simulink model "RefModel_SystemArchitecture"  (R2020a)
settings: Solver=ode1  StartTime=0.0  StopTime=inf  FixedStep=Ts_BigModel.Ts_base  MaxStep=Ts  RelTol=1e-3
undefined symbols (not defined in the file or in its folder): airspeed1, ENUM_SystemHealthStatus, ENUM_UavModel_Architecture, radar1, TASK_SET
libraries: simulink x1
settings Model: Creator=sl  LastModifiedBy=Administrator
settings DataIOCC: SaveOutput=off  SaveTime=off
settings OptimizationCC: DefaultParameterBehavior=Inlined  EnhancedBackFolding=on  PassReuseOutputArgsAs=Individual arguments  ZeroExternalMemoryAtStartup=off  ZeroInternalMemoryAtStartup=off  OptimizeBlockOrder=speed  DifferentSizesBufferReuse=on  OptimizationCustomize=off  EfficientTunableParamExpr=on
settings DebuggingCC: InheritedTsInSrcMsg=none  ParameterPrecisionLossMsg=none  ParameterTunabilityLossMsg=error  UnconnectedInputMsg=none  UnconnectedOutputMsg=none  UnconnectedLineMsg=none
settings HardwareCC: ProdBitPerPointer=32  ProdBitPerSizeT=32  ProdBitPerPtrDiffT=32  ProdLargestAtomicInteger=Long  ProdLargestAtomicFloat=Double  ProdWordSize=32  ProdHWDeviceType=ARM Compatible->ARM Cortex
settings ModelReferenceCC: ParallelModelReferenceMATLABWorkerInit=Copy Base Workspace  ModelReferenceNumInstancesAllowed=Single
settings SFSimCC: MATLABDynamicMemAlloc=off
settings RTWCC: SystemTargetFile=ert.tlc  GenCodeOnly=on  PackageGeneratedCodeAndArtifacts=on  TemplateMakefile=ert_default_tmf  GenerateReport=on  IncludeHyperlinkInReport=on  LaunchReport=on  GenerateTraceInfo=on  GenerateTraceReport=on  GenerateTraceReportSl=on  GenerateTraceReportSf=on  GenerateTraceReportEml=on
settings CodeAppCC: ForceParamTrailComments=on  IgnoreCustomStorageClasses=off  MaxIdLength=48  OperatorAnnotations=on  SimulinkDataObjDesc=on  SFDataObjDesc=on  MATLABFcnDesc=on  InsertBlockDesc=on  MATLABSourceComments=on
settings ERTTargetCC: TargetLangStandard=C99 (ISO)  GenerateSampleERTMain=on  LogVarNameModifier=none  SupportVariableSizeSignals=on  InlinedParameterPlacement=NonHierarchical  ERTCustomFileTemplate=example_file_process.tlc  ERTFilePackagingFormat=Compact

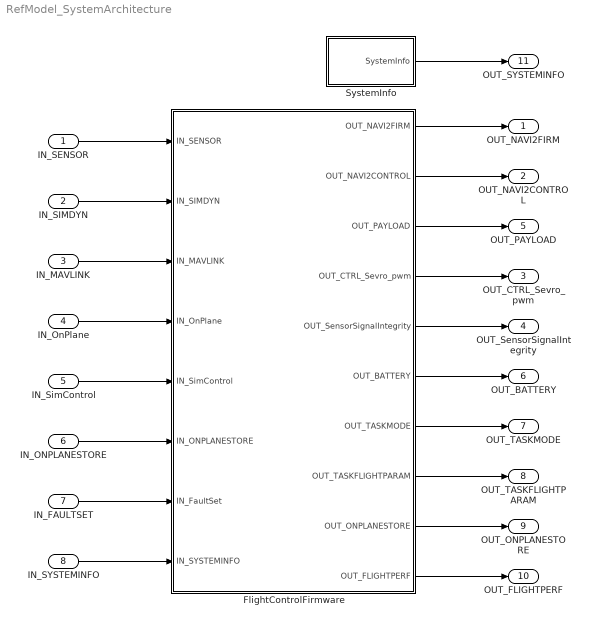
== system RefModel_SystemArchitecture ==
  IN_SENSOR : Inport  OutDataTypeStr=Bus: BUS_SENSOR
  IN_SIMDYN : Inport  Port=2  OutDataTypeStr=Bus: BUS_UAVDYN_FlightParam
  IN_MAVLINK : Inport  Port=3  OutDataTypeStr=Bus: BUS_MAVLINK_TO_FIRM  BusOutputAsStruct=on
  IN_OnPlane : Inport  Port=4  OutDataTypeStr=Bus: BUS_ONPLANE_FEEDBACK  BusOutputAsStruct=on
  IN_SimControl : Inport  Port=5  OutDataTypeStr=Bus: BUS_SIMCONTROL  BusOutputAsStruct=on
  IN_ONPLANESTORE : Inport  Port=6  OutDataTypeStr=Bus: BUS_ONPLANE_STORE  BusOutputAsStruct=on
  IN_FAULTSET : Inport  Port=7  OutDataTypeStr=Bus: BUS_SENSORFAULT_IN  BusOutputAsStruct=on
  IN_SYSTEMINFO : Inport  Port=8  OutDataTypeStr=Bus: BUS_SYSTEMINFO_INPUT  BusOutputAsStruct=on
  FlightControlFirmware : Subsystem
  SystemInfo : Subsystem
  " OUT_NAVI2FIRM" : Outport  OutDataTypeStr=Bus: BUS_NAVI_TO_FIRM
  OUT_NAVI2CONTROL : Outport  Port=2  OutDataTypeStr=Bus: BUS_TO_CONTROL
  OUT_CTRL_Sevro_pwm : Outport  Port=3  OutDataTypeStr=Bus: BUS_CTRL_Sevro_pwm  BusOutputAsStruct=on
  OUT_SensorSignalIntegrity : Outport  Port=4  OutDataTypeStr=Bus: BUS_NAVI_SensorSignalIntegrity
  OUT_PAYLOAD : Outport  Port=5  OutDataTypeStr=Bus: BUS_TASK_PAYLOAD  BusOutputAsStruct=on
  OUT_BATTERY : Outport  Port=6  OutDataTypeStr=Bus: BUS_TASK_BATTERY  BusOutputAsStruct=on
  OUT_TASKMODE : Outport  Port=7  OutDataTypeStr=Bus: BUS_TASK_PATH_OutParam
  OUT_TASKFLIGHTPARAM : Outport  Port=8  OutDataTypeStr=Bus: BUS_TASK_COMMON_OutParam
  OUT_ONPLANESTORE : Outport  Port=9  OutDataTypeStr=Bus: BUS_ONPLANE_STORE  BusOutputAsStruct=on
  OUT_FLIGHTPERF : Outport  Port=10  OutDataTypeStr=Bus: BUS_FLIGHTPERF_OUT
  " OUT_SYSTEMINFO" : Outport  Port=11  OutDataTypeStr=Bus: BUS_SYSTEMINFO  PortDimensions=1
  wires:
  IN_SIMDYN/1 -> FlightControlFirmware/2(IN_SIMDYN)
  FlightControlFirmware/4(OUT_CTRL_Sevro_pwm) -> OUT_CTRL_Sevro_pwm/1
  FlightControlFirmware/5(OUT_SensorSignalIntegrity) -> OUT_SensorSignalIntegrity/1
  FlightControlFirmware/1(OUT_NAVI2FIRM) -> " OUT_NAVI2FIRM"/1
  IN_OnPlane/1 -> FlightControlFirmware/4(IN_OnPlane)
  FlightControlFirmware/2(OUT_NAVI2CONTROL) -> OUT_NAVI2CONTROL/1
  IN_MAVLINK/1 -> FlightControlFirmware/3(IN_MAVLINK)
  FlightControlFirmware/3(OUT_PAYLOAD) -> OUT_PAYLOAD/1
  IN_SENSOR/1 -> FlightControlFirmware/1(IN_SENSOR)
  FlightControlFirmware/8(OUT_TASKFLIGHTPARAM) -> OUT_TASKFLIGHTPARAM/1
  FlightControlFirmware/7(OUT_TASKMODE) -> OUT_TASKMODE/1
  FlightControlFirmware/6(OUT_BATTERY) -> OUT_BATTERY/1
  IN_SimControl/1 -> FlightControlFirmware/5(IN_SimControl)
  IN_ONPLANESTORE/1 -> FlightControlFirmware/6(IN_ONPLANESTORE)
  FlightControlFirmware/9(OUT_ONPLANESTORE) -> OUT_ONPLANESTORE/1
  FlightControlFirmware/10(OUT_FLIGHTPERF) -> OUT_FLIGHTPERF/1
  IN_FAULTSET/1 -> FlightControlFirmware/7(IN_FaultSet)
  SystemInfo/1(SystemInfo) -> " OUT_SYSTEMINFO"/1
  IN_SYSTEMINFO/1 -> FlightControlFirmware/8(IN_SYSTEMINFO)

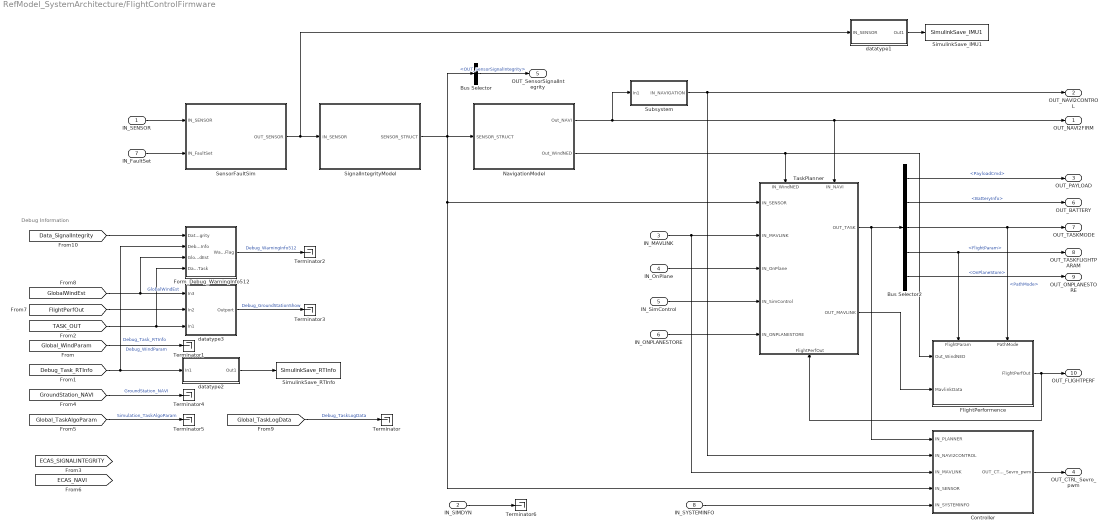
== system RefModel_SystemArchitecture/FlightControlFirmware ==
  note: Debug Information
  IN_SENSOR : Inport
  IN_SIMDYN : Inport  Port=2
  IN_MAVLINK : Inport  Port=3
  IN_OnPlane : Inport  Port=4
  IN_SimControl : Inport  Port=5
  IN_ONPLANESTORE : Inport  Port=6
  IN_FaultSet : Inport  Port=7
  IN_SYSTEMINFO : Inport  Port=8
  Bus Selector : BusSelector  OutputSignals=OUT_SensorSignalIntegrity
  Bus Selector2 : BusSelector  OutputSignals=PayloadCmd,BatteryInfo,PathMode,FlightParam,OnPlaneStore
  Controller : Subsystem
  FlightPerformence : Subsystem
      settings: PortSchema="{\"entries\":[{\"content\":{\"sides\":[{\"content\":{\"connectorIds\":[\"In1\",\"In2\"]},\"type\":\"ConnectorPlacement.EquallySpacedRectSide\",\"uuid\":\"433a6f53-ed4f-43c9-a2db-a1305bc564ee\"},{\"content\":{\"connectorIds\":[\"Out1\"],\"side\":\"RIGHT\"},\"type\":\"ConnectorPlacement.EquallySpacedRectSide\",\"uuid\":\"57435a5e-a27f-4849-b093-9cb5d83dc104\"},{\"content\":{\"connectorIds\":[\"In3\",\"In4\"],\"side\":\"TOP\"},\"type\":\"ConnectorPlacement.EquallySpacedRectSide\",\"uuid\":\"dceb23ba-b060-4a02-979b-0122130a3797\"}]},\"type\":\"ConnectorPlacement.EquallySpacedConnector\",\"uuid\":\"2c013d7c-89f2-45e4-826c-b5a23ebc63f7\"}],\"packageUris\":[\"http://schema.mathworks.com/mf0/Connector/19700101\"],\"version\":\"1.0\"}"
  Form_Debug_WarningInfo512 : Subsystem
  NavigationModel : Subsystem
  SensorFaultSim : Subsystem
  SignalIntegrityModel : Subsystem
  SimulinkSave_IMU1 : ToWorkspace  VariableName=SimulinkSave_IMU1  SaveFormat=Structure With Time  SampleTime=-1
  SimulinkSave_RTInfo : ToWorkspace  VariableName=SimulinkSave_RTInfo  SaveFormat=Structure With Time  SampleTime=-1
  Subsystem : Subsystem
  TaskPlanner : Subsystem
      settings: PortSchema="{\"entries\":[{\"content\":{\"sides\":[{\"content\":{\"connectorIds\":[\"In1\",\"In2\",\"In3\",\"In4\",\"In5\"]},\"type\":\"ConnectorPlacement.EquallySpacedRectSide\",\"uuid\":\"cf788447-cee3-4dc7-a19e-d1c3b675d866\"},{\"content\":{\"connectorIds\":[\"Out1\",\"Out2\"],\"side\":\"RIGHT\"},\"type\":\"ConnectorPlacement.EquallySpacedRectSide\",\"uuid\":\"de502817-2f17-4bc5-82c1-7b7d96fa5a18\"},{\"content\":{\"connectorIds\":[\"In6\",\"In7\"],\"side\":\"TOP\"},\"type\":\"ConnectorPlacement.EquallySpacedRectSide\",\"uuid\":\"c2c5d609-21c0-4e27-8129-13e054f6685c\"},{\"content\":{\"connectorIds\":[\"In8\"],\"side\":\"BOTTOM\"},\"type\":\"ConnectorPlacement.EquallySpacedRectSide\",\"uuid\":\"4fcd6bd9-9831-4959-9cb5-0a694e5ed564\"}]},\"type\":\"ConnectorPlacement.EquallySpacedConnector\",\"uuid\":\"8f2d23fd-8a63-42f8-87e9-439a9ee38a82\"}],\"packageUris\":[\"http://schema.mathworks.com/mf0/Connector/19700101\"],\"version\":\"1.0\"}"
  Terminator{,1..6} (7 alike) : Terminator
  datatype1 : Subsystem
  datatype2 : Subsystem
  datatype3 : Subsystem
  OUT_NAVI2FIRM : Outport
  OUT_NAVI2CONTROL : Outport  Port=2
  OUT_PAYLOAD : Outport  Port=3
  OUT_CTRL_Sevro_pwm : Outport  Port=4
  OUT_SensorSignalIntegrity : Outport  Port=5  OutDataTypeStr=Bus: BUS_NAVI_SensorSignalIntegrity
  OUT_BATTERY : Outport  Port=6
  OUT_TASKMODE : Outport  Port=7
  OUT_TASKFLIGHTPARAM : Outport  Port=8
  OUT_ONPLANESTORE : Outport  Port=9
  OUT_FLIGHTPERF : Outport  Port=10
  wires:
  Subsystem/1(IN_NAVIGATION) -> Controller/2(IN_NAVI2CONTROL), OUT_NAVI2CONTROL/1
  IN_MAVLINK/1 -> TaskPlanner/2(IN_MAVLINK), Controller/3(IN_MAVLINK)
  TaskPlanner/1(OUT_TASK) -> Controller/1(IN_PLANNER), Bus Selector2/1
  Controller/1(OUT_CTRL_Sevro_pwm) -> OUT_CTRL_Sevro_pwm/1
  IN_SIMDYN/1 -> Terminator6/1
  NavigationModel/1(Out_NAVI) -> OUT_NAVI2FIRM/1, TaskPlanner/7(IN_NAVI), Subsystem/1(In1)
  Bus Selector/1 -> OUT_SensorSignalIntegrity/1  "<OUT_SensorSignalIntegrity>"
  SignalIntegrityModel/1(SENSOR_STRUCT) -> Controller/4(IN_SENSOR), TaskPlanner/1(IN_SENSOR), NavigationModel/1(SENSOR_STRUCT), Bus Selector/1
  IN_OnPlane/1 -> TaskPlanner/3(IN_OnPlane)
  IN_SimControl/1 -> TaskPlanner/4(IN_SimControl)
  [Debug_Task_RTInfo] -> Form_Debug_WarningInfo512/2(Debug_Task_RTInfo), datatype2/1(In1)  "Debug_Task_RTInfo"
  [GroundStation_NAVI] -> Terminator4/1  "GroundStation_NAVI"
  Bus Selector2/1 -> OUT_PAYLOAD/1  "<PayloadCmd>"
  Bus Selector2/2 -> OUT_BATTERY/1  "<BatteryInfo>"
  Bus Selector2/3 -> OUT_TASKMODE/1, FlightPerformence/4(PathMode)  "<PathMode>"
  Bus Selector2/4 -> OUT_TASKFLIGHTPARAM/1, FlightPerformence/3(FlightParam)  "<FlightParam>"
  datatype1/1(Out1) -> SimulinkSave_IMU1/1
  [Global_TaskAlgoParam] -> Terminator5/1  "Simulation_TaskAlgoParam"
  Bus Selector2/5 -> OUT_ONPLANESTORE/1  "<OnPlaneStore>"
  IN_ONPLANESTORE/1 -> TaskPlanner/5(IN_ONPLANESTORE)
  datatype2/1(Out1) -> SimulinkSave_RTInfo/1
  [Global_WindParam] -> Terminator1/1  "Debug_WindParam"
  [TASK_OUT] -> Form_Debug_WarningInfo512/4(Data_Task), datatype3/3(In1)
  datatype3/1(Outport) -> Terminator3/1  "Debug_GroundStationShow"
  FlightPerformence/1(FlightPerfOut) -> TaskPlanner/8(FlightPerfOut), OUT_FLIGHTPERF/1
  [FlightPerfOut] -> datatype3/2(In2)
  SensorFaultSim/1(OUT_SENSOR) -> datatype1/1(IN_SENSOR), SignalIntegrityModel/1(IN_SENSOR)
  IN_SENSOR/1 -> SensorFaultSim/1(IN_SENSOR)
  IN_FaultSet/1 -> SensorFaultSim/2(IN_FaultSet)
  [GlobalWindEst] -> Form_Debug_WarningInfo512/3(GlobalWindEst), datatype3/1(In3)  "GlobalWindEst"
  Form_Debug_WarningInfo512/1(WarningFlag) -> Terminator2/1  "Debug_WarningInfo512"
  NavigationModel/2(Out_WindNED) -> FlightPerformence/1(Out_WindNED), TaskPlanner/6(IN_WindNED)
  TaskPlanner/2(OUT_MAVLINK) -> FlightPerformence/2(MavlinkData)
  [Global_TaskLogData] -> Terminator/1  "Debug_TaskLogData"
  [Data_SignalIntegrity] -> Form_Debug_WarningInfo512/1(Data_SignalIntegrity)
  IN_SYSTEMINFO/1 -> Controller/5(IN_SYSTEMINFO)

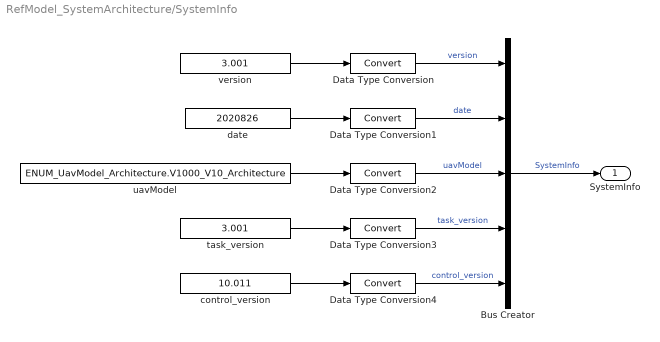
== system RefModel_SystemArchitecture/SystemInfo ==
  Bus Creator : BusCreator  Inputs=5
  Data Type Conversion{,1..4} (5 alike) : DataTypeConversion
  control_version : Constant  Value=10.011
  date : Constant  Value=2020826
  task_version : Constant  Value=3.001
  uavModel : Constant  Value=ENUM_UavModel_Architecture.V1000_V10_Architecture
  version : Constant  Value=3.001
  SystemInfo : Outport
  wires:
  version/1 -> Data Type Conversion/1
  Bus Creator/1 -> SystemInfo/1  "SystemInfo"
  date/1 -> Data Type Conversion1/1
  Data Type Conversion/1 -> Bus Creator/1  "version"
  Data Type Conversion1/1 -> Bus Creator/2  "date"
  uavModel/1 -> Data Type Conversion2/1
  Data Type Conversion2/1 -> Bus Creator/3  "uavModel"
  task_version/1 -> Data Type Conversion3/1
  control_version/1 -> Data Type Conversion4/1
  Data Type Conversion3/1 -> Bus Creator/4  "task_version"
  Data Type Conversion4/1 -> Bus Creator/5  "control_version"

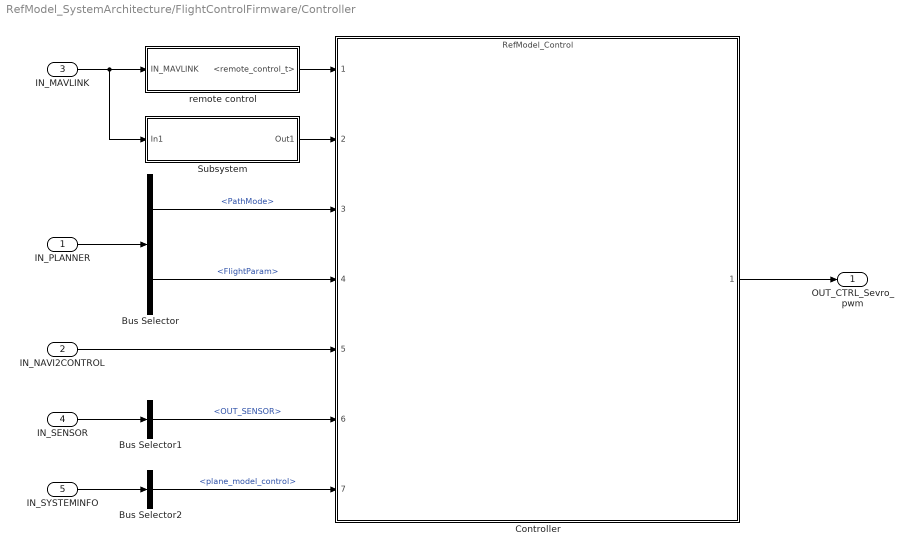
== system RefModel_SystemArchitecture/FlightControlFirmware/Controller ==
  IN_PLANNER : Inport
  IN_NAVI2CONTROL : Inport  Port=2
  IN_MAVLINK : Inport  Port=3  BusOutputAsStruct=on
  IN_SENSOR : Inport  Port=4
  IN_SYSTEMINFO : Inport  Port=5
  Bus Selector : BusSelector  OutputSignals=PathMode,FlightParam
  Bus Selector1 : BusSelector  OutputSignals=OUT_SENSOR
  Bus Selector2 : BusSelector  OutputSignals=plane_model_control
  Controller : ModelReference  ModelNameDialog=RefModel_Control.slx  SimulationMode=Normal  CachedPortDiscreteRates=[0.04]  ModelReferenceVersion=1.998
  Subsystem : Subsystem
  remote control : Subsystem
  OUT_CTRL_Sevro_pwm : Outport
  wires:
  Controller/1 -> OUT_CTRL_Sevro_pwm/1
  IN_NAVI2CONTROL/1 -> Controller/5
  IN_SENSOR/1 -> Bus Selector1/1
  IN_PLANNER/1 -> Bus Selector/1
  Bus Selector/1 -> Controller/3  "<PathMode>"
  Bus Selector/2 -> Controller/4  "<FlightParam>"
  remote control/1(<remote_control_t>) -> Controller/1
  IN_MAVLINK/1 -> Subsystem/1(In1), remote control/1(IN_MAVLINK)
  Subsystem/1(Out1) -> Controller/2
  IN_SYSTEMINFO/1 -> Bus Selector2/1
  Bus Selector1/1 -> Controller/6  "<OUT_SENSOR>"
  Bus Selector2/1 -> Controller/7  "<plane_model_control>"

== system RefModel_SystemArchitecture/FlightControlFirmware/FlightPerformence ==
  Out_WindNED : Inport
  MavlinkData : Inport  Port=2
  FlightParam : Inport  Port=3
  PathMode : Inport  Port=4
  FlightPerformance : ModelReference  ModelNameDialog=RefModel_FlightPerf.slx  SimulationMode=Normal  CachedPortDiscreteRates=[0.04]  ModelReferenceVersion=1.3475
  FlightPerfOut : Outport
  tag scope: FlightPerfOut=global
  wires:
  FlightParam/1 -> FlightPerformance/2
  PathMode/1 -> FlightPerformance/1
  MavlinkData/1 -> FlightPerformance/3
  FlightPerformance/1 -> [FlightPerfOut], FlightPerfOut/1
  Out_WindNED/1 -> FlightPerformance/4

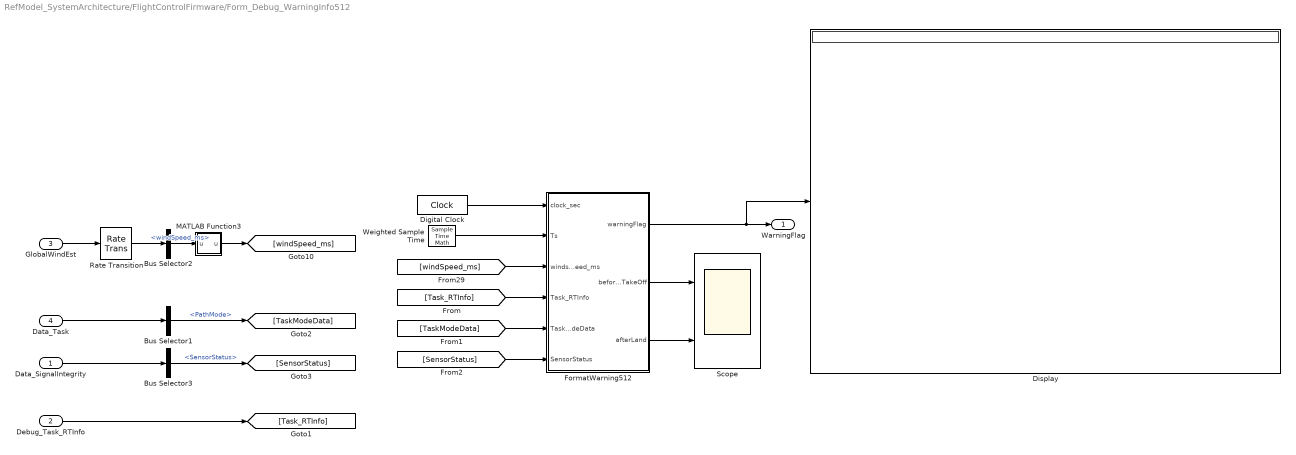
== system RefModel_SystemArchitecture/FlightControlFirmware/Form_Debug_WarningInfo512 ==
  Data_SignalIntegrity : Inport
  Debug_Task_RTInfo : Inport  Port=2
  GlobalWindEst : Inport  Port=3
  Data_Task : Inport  Port=4
  Bus Selector1 : BusSelector  OutputSignals=PathMode
  Bus Selector2 : BusSelector  OutputSignals=windSpeed_ms
  Bus Selector3 : BusSelector  OutputSignals=SensorStatus
  Digital Clock : DigitalClock  SampleTime=-1
  Display : Display
  FormatWarning512 : MATLAB Function  TreatAsAtomicUnit=on
  MATLAB Function3 : MATLAB Function  TreatAsAtomicUnit=on
  Rate Transition : RateTransition
  Scope : Scope  NumInputPorts=2
  Weighted Sample Time : SampleTimeMath  TsampMathOp=Ts Only
  WarningFlag : Outport
  wires:
  [windSpeed_ms] -> FormatWarning512/3(windspeed_ms)
  MATLAB Function3/1(u) -> [windSpeed_ms]
  GlobalWindEst/1 -> Rate Transition/1
  Bus Selector2/1 -> MATLAB Function3/1("u ")  "<windSpeed_ms>"
  Rate Transition/1 -> Bus Selector2/1
  FormatWarning512/1(warningFlag) -> Display/1, WarningFlag/1
  Debug_Task_RTInfo/1 -> [Task_RTInfo]
  [Task_RTInfo] -> FormatWarning512/4(Task_RTInfo)
  Data_Task/1 -> Bus Selector1/1
  Bus Selector1/1 -> [TaskModeData]  "<PathMode>"
  [TaskModeData] -> FormatWarning512/5(TaskModeData)
  Data_SignalIntegrity/1 -> Bus Selector3/1
  Bus Selector3/1 -> [SensorStatus]  "<SensorStatus>"
  [SensorStatus] -> FormatWarning512/6(SensorStatus)
  Weighted Sample Time/1 -> FormatWarning512/2(Ts)
  Digital Clock/1 -> FormatWarning512/1(clock_sec)
  FormatWarning512/2(beforeTakeOff) -> Scope/1
  FormatWarning512/3(afterLand) -> Scope/2

== system RefModel_SystemArchitecture/FlightControlFirmware/NavigationModel ==
  SENSOR_STRUCT : Inport
  Bus Selector1 : BusSelector  OutputSignals=OUT_SENSOR,OUT_SensorSignalIntegrity
  NavigationModel : ModelReference  ModelNameDialog=RefModel_Navfilter  SimulationMode=Normal  CachedPortDiscreteRates=[0.004]  ModelReferenceVersion=1.1444
  Terminator2 : Terminator
  Out_NAVI : Outport
  Out_WindNED : Outport  Port=2
  tag scope: ECAS_NAVI=global, GlobalWindEst=global
  wires:
  NavigationModel/1 -> Out_NAVI/1
  Bus Selector1/1 -> NavigationModel/1  "<OUT_SENSOR>"
  Bus Selector1/2 -> NavigationModel/2  "<OUT_SensorSignalIntegrity>"
  SENSOR_STRUCT/1 -> Bus Selector1/1
  NavigationModel/4 -> Out_WindNED/1, [GlobalWindEst]
  NavigationModel/3 -> Terminator2/1
  NavigationModel/2 -> [ECAS_NAVI]

== system RefModel_SystemArchitecture/FlightControlFirmware/SensorFaultSim ==
  IN_SENSOR : Inport
  IN_FaultSet : Inport  Port=2
  SignalFaultModel : ModelReference  DisableCoverage=on  ModelNameDialog=RefModel_SensorFault.slx  SimulationMode=Normal  ModelReferenceVersion=1.387
  OUT_SENSOR : Outport
  wires:
  IN_SENSOR/1 -> SignalFaultModel/1
  IN_FaultSet/1 -> SignalFaultModel/2
  SignalFaultModel/1 -> OUT_SENSOR/1

== system RefModel_SystemArchitecture/FlightControlFirmware/SignalIntegrityModel ==
  IN_SENSOR : Inport
  Bus Creator : BusCreator  Inputs=2
  NavigationModel : ModelReference  ModelNameDialog=RefModel_SignalIntegrity  SimulationMode=Normal  CachedPortDiscreteRates=[0.004]  ModelReferenceVersion=1.653
  SENSOR_STRUCT : Outport
  tag scope: Data_SignalIntegrity=global, ECAS_SIGNALINTEGRITY=global
  wires:
  IN_SENSOR/1 -> NavigationModel/1
  NavigationModel/2 -> [Data_SignalIntegrity], Bus Creator/2  "OUT_SensorSignalIntegrity"
  NavigationModel/1 -> Bus Creator/1  "OUT_SENSOR"
  Bus Creator/1 -> SENSOR_STRUCT/1
  NavigationModel/3 -> [ECAS_SIGNALINTEGRITY]

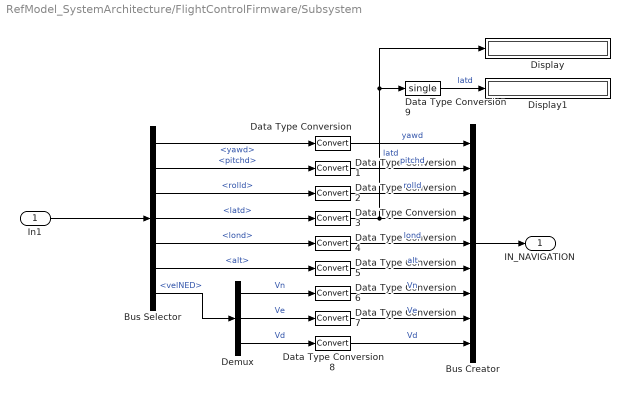
== system RefModel_SystemArchitecture/FlightControlFirmware/Subsystem ==
  In1 : Inport
  Bus Creator : BusCreator  Inputs=9
  Bus Selector : BusSelector  OutputSignals=yawd,pitchd,rolld,latd,lond,alt,velNED
  Data Type Conversion{,1..8} (9 alike) : DataTypeConversion
  Data Type Conversion9 : DataTypeConversion  OutDataTypeStr=single
  Demux : Demux  Outputs=3
  Display : Display
  Display1 : Display
  IN_NAVIGATION : Outport
  wires:
  In1/1 -> Bus Selector/1
  Bus Selector/7 -> Demux/1  "<velNED>"
  Bus Selector/1 -> Data Type Conversion/1  "<yawd>"
  Bus Selector/2 -> Data Type Conversion1/1  "<pitchd>"
  Bus Selector/3 -> Data Type Conversion2/1  "<rolld>"
  Bus Selector/4 -> Data Type Conversion3/1  "<latd>"
  Bus Selector/5 -> Data Type Conversion4/1  "<lond>"
  Bus Selector/6 -> Data Type Conversion5/1  "<alt>"
  Demux/3 -> Data Type Conversion8/1  "Vd"
  Demux/2 -> Data Type Conversion7/1  "Ve"
  Demux/1 -> Data Type Conversion6/1  "Vn"
  Bus Creator/1 -> IN_NAVIGATION/1
  Data Type Conversion/1 -> Bus Creator/1  "yawd"
  Data Type Conversion1/1 -> Bus Creator/2  "pitchd"
  Data Type Conversion2/1 -> Bus Creator/3  "rolld"
  Data Type Conversion3/1 -> Data Type Conversion9/1, Display/1, Bus Creator/4  "latd"
  Data Type Conversion4/1 -> Bus Creator/5  "lond"
  Data Type Conversion6/1 -> Bus Creator/7  "Vn"
  Data Type Conversion5/1 -> Bus Creator/6  "alt"
  Data Type Conversion7/1 -> Bus Creator/8  "Ve"
  Data Type Conversion8/1 -> Bus Creator/9  "Vd"
  Data Type Conversion9/1 -> Display1/1  "latd"

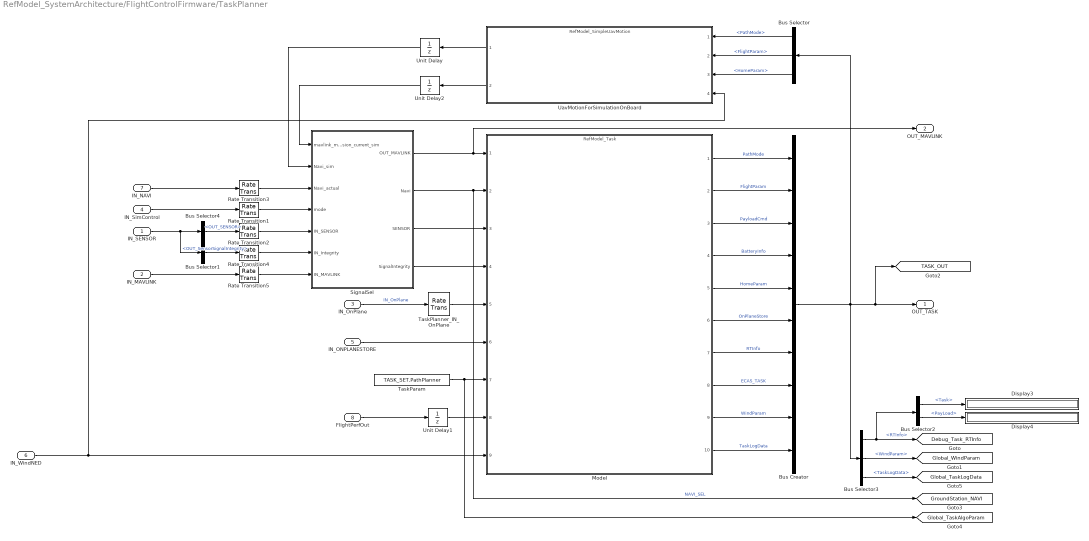
== system RefModel_SystemArchitecture/FlightControlFirmware/TaskPlanner ==
  IN_SENSOR : Inport
  IN_MAVLINK : Inport  Port=2
  IN_OnPlane : Inport  Port=3  BusOutputAsStruct=on
  IN_SimControl : Inport  Port=4
  IN_ONPLANESTORE : Inport  Port=5  BusOutputAsStruct=on
  IN_WindNED : Inport  Port=6
  IN_NAVI : Inport  Port=7
  FlightPerfOut : Inport  Port=8
  Bus Creator : BusCreator  Inputs=10
  Bus Selector : BusSelector  OutputSignals=PathMode,FlightParam,HomeParam
  Bus Selector1 : BusSelector  OutputSignals=OUT_SensorSignalIntegrity
  Bus Selector2 : BusSelector  OutputSignals=Task,PayLoad
  Bus Selector3 : BusSelector  OutputSignals=RTInfo,WindParam,TaskLogData
  Bus Selector4 : BusSelector  OutputSignals=OUT_SENSOR
  Display3 : Display
  Display4 : Display
  Model : ModelReference  ModelNameDialog=RefModel_Task.slx  SimulationMode=Normal  CachedPortDiscreteRates=[0.04]  ModelReferenceVersion=1.5844
  Rate Transition{1..5} (5 alike) : RateTransition
  SignalSel : Subsystem
  TaskParam : Constant  Value=TASK_SET.PathPlanner  OutDataTypeStr=Bus: BUS_TASK_PATH_AlgoParam
  TaskPlanner_IN_OnPlane : RateTransition
  UavMotionForSimulationOnBoard : ModelReference  ModelNameDialog=RefModel_SimpleUavMotion.slx  SimulationMode=Normal  CachedPortDiscreteRates=[0.04]  ModelReferenceVersion=1.1025
  Unit Delay : UnitDelay  SampleTime=-1  HasFrameUpgradeWarning=on
  Unit Delay1 : UnitDelay  SampleTime=-1  HasFrameUpgradeWarning=on
  Unit Delay2 : UnitDelay  SampleTime=-1  HasFrameUpgradeWarning=on
  OUT_TASK : Outport
  OUT_MAVLINK : Outport  Port=2
  tag scope: Debug_Task_RTInfo=global, Global_TaskAlgoParam=global, Global_TaskLogData=global, Global_WindParam=global, GroundStation_NAVI=global, TASK_OUT=global
  wires:
  SignalSel/1(OUT_MAVLINK) -> OUT_MAVLINK/1, Model/1
  SignalSel/3(SENSOR) -> Model/3
  IN_SENSOR/1 -> Bus Selector1/1, Bus Selector4/1
  SignalSel/4(SignalIntegrity) -> Model/4
  IN_OnPlane/1 -> TaskPlanner_IN_OnPlane/1  "IN_OnPlane"
  Model/1 -> Bus Creator/1  "PathMode"
  Model/2 -> Bus Creator/2  "FlightParam"
  Model/3 -> Bus Creator/3  "PayloadCmd"
  Model/4 -> Bus Creator/4  "BatteryInfo"
  Model/5 -> Bus Creator/5  "HomeParam"
  TaskPlanner_IN_OnPlane/1 -> Model/5
  Model/7 -> Bus Creator/7  "RTInfo"
  UavMotionForSimulationOnBoard/1 -> Unit Delay/1
  IN_NAVI/1 -> Rate Transition3/1
  IN_SimControl/1 -> Rate Transition1/1
  SignalSel/2(Navi) -> Model/2, [GroundStation_NAVI]  "NAVI_SEL"
  Unit Delay/1 -> SignalSel/2(Navi_sim)
  Bus Creator/1 -> [TASK_OUT], OUT_TASK/1, Bus Selector3/1, Bus Selector/1
  Bus Selector4/1 -> Rate Transition2/1  "<OUT_SENSOR>"
  Bus Selector1/1 -> Rate Transition4/1  "<OUT_SensorSignalIntegrity>"
  IN_ONPLANESTORE/1 -> Model/6
  Model/8 -> Bus Creator/8  "ECAS_TASK"
  Model/6 -> Bus Creator/6  "OnPlaneStore"
  Model/9 -> Bus Creator/9  "WindParam"
  Rate Transition3/1 -> SignalSel/3(Navi_actual)
  Rate Transition1/1 -> SignalSel/4(mode)
  Rate Transition2/1 -> SignalSel/5(IN_SENSOR)
  Rate Transition4/1 -> SignalSel/6(IN_Integrity)
  TaskParam/1 -> Model/7, [Global_TaskAlgoParam]
  FlightPerfOut/1 -> Unit Delay1/1
  Unit Delay1/1 -> Model/8
  IN_WindNED/1 -> UavMotionForSimulationOnBoard/4, Model/9
  UavMotionForSimulationOnBoard/2 -> Unit Delay2/1
  IN_MAVLINK/1 -> Rate Transition5/1
  Rate Transition5/1 -> SignalSel/7(IN_MAVLINK)
  Unit Delay2/1 -> SignalSel/1(mavlink_msg_mission_current_sim)
  Model/10 -> Bus Creator/10  "TaskLogData"
  Bus Selector/1 -> UavMotionForSimulationOnBoard/1  "<PathMode>"
  Bus Selector/2 -> UavMotionForSimulationOnBoard/2  "<FlightParam>"
  Bus Selector/3 -> UavMotionForSimulationOnBoard/3  "<HomeParam>"
  Bus Selector2/2 -> Display4/1  "<PayLoad>"
  Bus Selector2/1 -> Display3/1  "<Task>"
  Bus Selector3/1 -> Bus Selector2/1, [Debug_Task_RTInfo]  "<RTInfo>"
  Bus Selector3/2 -> [Global_WindParam]  "<WindParam>"
  Bus Selector3/3 -> [Global_TaskLogData]  "<TaskLogData>"

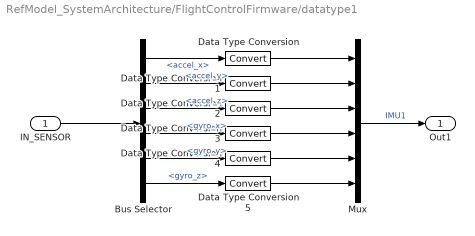
== system RefModel_SystemArchitecture/FlightControlFirmware/datatype1 ==
  IN_SENSOR : Inport
  Bus Selector : BusSelector  OutputSignals=IMU1.accel_x,IMU1.accel_y,IMU1.accel_z,IMU1.gyro_x,IMU1.gyro_y,IMU1.gyro_z
  Data Type Conversion{,1..5} (6 alike) : DataTypeConversion
  Mux : Mux  Inputs=6
  Out1 : Outport
  wires:
  IN_SENSOR/1 -> Bus Selector/1
  Bus Selector/1 -> Data Type Conversion/1  "<accel_x>"
  Bus Selector/2 -> Data Type Conversion1/1  "<accel_y>"
  Bus Selector/3 -> Data Type Conversion2/1  "<accel_z>"
  Bus Selector/4 -> Data Type Conversion3/1  "<gyro_x>"
  Bus Selector/5 -> Data Type Conversion4/1  "<gyro_y>"
  Bus Selector/6 -> Data Type Conversion5/1  "<gyro_z>"
  Mux/1 -> Out1/1  "IMU1"
  Data Type Conversion/1 -> Mux/1
  Data Type Conversion1/1 -> Mux/2
  Data Type Conversion2/1 -> Mux/3
  Data Type Conversion3/1 -> Mux/4
  Data Type Conversion4/1 -> Mux/5
  Data Type Conversion5/1 -> Mux/6

== system RefModel_SystemArchitecture/FlightControlFirmware/datatype2 ==
  In1 : Inport
  Bus Selector : BusSelector  OutputSignals=Task,PayLoad,GSCmd,Warning
  Data Type Conversion{,1..3} (4 alike) : DataTypeConversion
  Mux : Mux
  Out1 : Outport
  wires:
  In1/1 -> Bus Selector/1
  Bus Selector/1 -> Data Type Conversion/1  "<Task>"
  Bus Selector/2 -> Data Type Conversion1/1  "<PayLoad>"
  Mux/1 -> Out1/1  "IMU1"
  Data Type Conversion/1 -> Mux/1
  Data Type Conversion1/1 -> Mux/2
  Bus Selector/3 -> Data Type Conversion2/1  "<GSCmd>"
  Bus Selector/4 -> Data Type Conversion3/1  "<Warning>"
  Data Type Conversion2/1 -> Mux/3
  Data Type Conversion3/1 -> Mux/4

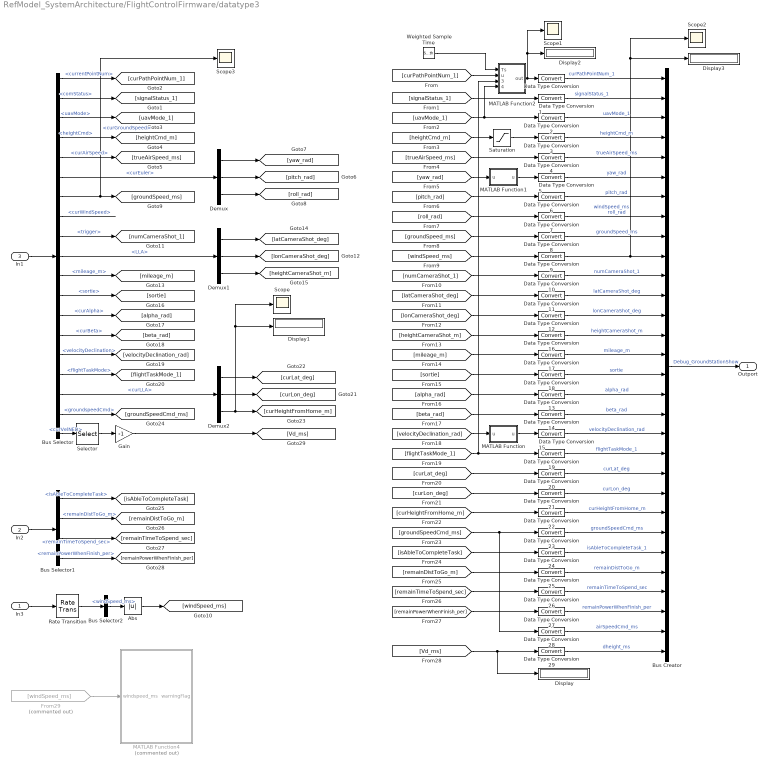
== system RefModel_SystemArchitecture/FlightControlFirmware/datatype3 ==
  In3 : Inport
  In2 : Inport  Port=2
  In1 : Inport  Port=3
  Abs : Abs
  Bus Creator : BusCreator  Inputs=30  OutDataTypeStr=Bus: BUS_GROUNDSTATION_SHOW  NonVirtualBus=on
  Bus Selector : BusSelector  OutputSignals=PathMode.currentPointNum,PathMode.comStatus,PathMode.uavMode,PathMode.heightCmd,FlightParam.curAirSpeed,FlightParam.curEuler,FlightParam.curGroundSpeed,FlightParam.curWindSpeed,PayloadCmd.CAMERA.trigger,PayloadCmd.CAMERA.LLA,OnPlaneStore.mileage_m,OnPlaneStore.Number.sortie,FlightParam.curAlpha,FlightParam.curBeta,FlightParam.velocityDeclination,PathMode.flightTaskMode,FlightParam.curLLA,PathMode.groundspeedCmd,FlightParam.curVelNED
  Bus Selector1 : BusSelector  OutputSignals=isAbleToCompleteTask,remainDistToGo_m,remainTimeToSpend_sec,remainPowerWhenFinish_per
  Bus Selector2 : BusSelector  OutputSignals=windSpeed_ms
  Data Type Conversion{,1..29} (30 alike) : DataTypeConversion
  Demux : Demux  Outputs=3
  Demux1 : Demux  Outputs=3
  Demux2 : Demux  Outputs=3
  Display{,1..3} (4 alike) : Display
  From29 : From  Commented=on  GotoTag=windSpeed_ms
  Gain : Gain  Gain=-1
  MATLAB Function : MATLAB Function  TreatAsAtomicUnit=on
  MATLAB Function1 : MATLAB Function  TreatAsAtomicUnit=on
  MATLAB Function2 : MATLAB Function  TreatAsAtomicUnit=on
  MATLAB Function4 : MATLAB Function  Commented=on  TreatAsAtomicUnit=on
  Rate Transition : RateTransition
  Saturation : Saturate  UpperLimit=inf  LowerLimit=0
  Scope{,1..3} (4 alike) : Scope
  Selector : Selector  InputPortWidth=3  IndexOptions=Index vector (dialog)  Indices=[3]  OutputSizes=1
  Weighted Sample Time : SampleTimeMath  TsampMathOp=Ts Only
  Outport : Outport  OutDataTypeStr=Bus: BUS_GROUNDSTATION_SHOW
  wires:
  In1/1 -> Bus Selector/1
  Bus Selector/10 -> Demux1/1  "<LLA>"
  Bus Selector/9 -> [numCameraShot_1]  "<trigger>"
  Bus Selector/11 -> [mileage_m]  "<mileage_m>"
  Bus Selector/8 -> ?  "<curWindSpeed>"
  Bus Selector/12 -> [sortie]  "<sortie>"
  Bus Selector/7 -> Scope3/1, [groundSpeed_ms]  "<curGroundSpeed>"
  Bus Selector/6 -> Demux/1  "<curEuler>"
  Bus Selector/5 -> [trueAirSpeed_ms]  "<curAirSpeed>"
  Bus Selector/4 -> [heightCmd_m]  "<heightCmd>"
  Bus Selector/3 -> [uavMode_1]  "<uavMode>"
  Bus Selector/2 -> [signalStatus_1]  "<comStatus>"
  Bus Selector/1 -> [curPathPointNum_1]  "<currentPointNum>"
  Data Type Conversion/1 -> Bus Creator/1  "curPathPointNum_1"
  Data Type Conversion1/1 -> Bus Creator/2  "signalStatus_1"
  Data Type Conversion2/1 -> Bus Creator/3  "uavMode_1"
  Data Type Conversion3/1 -> Bus Creator/4  "heightCmd_m"
  Data Type Conversion4/1 -> Bus Creator/5  "trueAirSpeed_ms"
  Data Type Conversion5/1 -> Bus Creator/6  "yaw_rad"
  Data Type Conversion6/1 -> Bus Creator/7  "pitch_rad"
  Data Type Conversion7/1 -> Bus Creator/8  "roll_rad"
  Data Type Conversion8/1 -> Bus Creator/9  "groundSpeed_ms"
  Data Type Conversion9/1 -> Scope2/1, Display3/1, Bus Creator/10  "windSpeed_ms"
  Data Type Conversion10/1 -> Bus Creator/11  "numCameraShot_1"
  Data Type Conversion11/1 -> Bus Creator/12  "latCameraShot_deg"
  Demux/2 -> [pitch_rad]
  Demux/1 -> [yaw_rad]
  Demux/3 -> [roll_rad]
  Demux1/3 -> [heightCameraShot_m]
  Demux1/1 -> [latCameraShot_deg]
  Demux1/2 -> [lonCameraShot_deg]
  [curPathPointNum_1] -> MATLAB Function2/2(u)
  [signalStatus_1] -> Data Type Conversion1/1
  [uavMode_1] -> MATLAB Function2/4(uavmode), Data Type Conversion2/1
  [heightCmd_m] -> Saturation/1
  [trueAirSpeed_ms] -> Data Type Conversion4/1
  [yaw_rad] -> MATLAB Function1/1("u ")
  [pitch_rad] -> Data Type Conversion6/1
  [roll_rad] -> Data Type Conversion7/1
  [groundSpeed_ms] -> Data Type Conversion8/1
  [windSpeed_ms] -> Data Type Conversion9/1
  [numCameraShot_1] -> Data Type Conversion10/1
  [latCameraShot_deg] -> Data Type Conversion11/1
  [lonCameraShot_deg] -> Data Type Conversion12/1
  Data Type Conversion12/1 -> Bus Creator/13  "lonCameraShot_deg"
  [heightCameraShot_m] -> Data Type Conversion16/1
  Data Type Conversion16/1 -> Bus Creator/14  "heightCameraShot_m"
  [mileage_m] -> Data Type Conversion17/1
  Data Type Conversion17/1 -> Bus Creator/15  "mileage_m"
  [sortie] -> Data Type Conversion18/1
  Data Type Conversion18/1 -> Bus Creator/16  "sortie"
  Bus Selector/13 -> [alpha_rad]  "<curAlpha>"
  Bus Selector/14 -> [beta_rad]  "<curBeta>"
  [alpha_rad] -> Data Type Conversion13/1
  Data Type Conversion13/1 -> Bus Creator/17  "alpha_rad"
  [beta_rad] -> Data Type Conversion14/1
  Data Type Conversion14/1 -> Bus Creator/18  "beta_rad"
  Data Type Conversion15/1 -> Bus Creator/19  "velocityDeclination_rad"
  Data Type Conversion19/1 -> Bus Creator/20  "flightTaskMode_1"
  Bus Creator/1 -> Outport/1  "Debug_GroundStationShow"
  Bus Selector/15 -> [velocityDeclination_rad]  "<velocityDeclination>"
  [velocityDeclination_rad] -> MATLAB Function/1("u ")
  Bus Selector/16 -> [flightTaskMode_1]  "<flightTaskMode>"
  [flightTaskMode_1] -> MATLAB Function2/3(taskmode), Data Type Conversion19/1
  MATLAB Function/1(u) -> Data Type Conversion15/1
  MATLAB Function1/1(u) -> Data Type Conversion5/1
  Bus Selector/17 -> Demux2/1  "<curLLA>"
  Demux2/2 -> [curLon_deg]
  Demux2/1 -> [curLat_deg]
  [curLon_deg] -> Data Type Conversion21/1
  [curLat_deg] -> Data Type Conversion20/1
  [curHeightFromHome_m] -> Data Type Conversion22/1
  Data Type Conversion20/1 -> Bus Creator/21  "curLat_deg"
  Data Type Conversion21/1 -> Bus Creator/22  "curLon_deg"
  Data Type Conversion22/1 -> Bus Creator/23  "curHeightFromHome_m"
  Bus Selector/18 -> [groundSpeedCmd_ms]  "<groundspeedCmd>"
  [groundSpeedCmd_ms] -> Data Type Conversion28/1, Data Type Conversion23/1
  Data Type Conversion23/1 -> Bus Creator/24  "groundSpeedCmd_ms"
  In2/1 -> Bus Selector1/1
  Bus Selector1/3 -> [remainTimeToSpend_sec]  "<remainTimeToSpend_sec>"
  Bus Selector1/2 -> [remainDistToGo_m]  "<remainDistToGo_m>"
  Bus Selector1/4 -> [remainPowerWhenFinish_per]  "<remainPowerWhenFinish_per>"
  Bus Selector1/1 -> [isAbleToCompleteTask]  "<isAbleToCompleteTask>"
  [isAbleToCompleteTask] -> Data Type Conversion24/1
  [remainDistToGo_m] -> Data Type Conversion25/1
  [remainTimeToSpend_sec] -> Data Type Conversion26/1
  [remainPowerWhenFinish_per] -> Data Type Conversion27/1
  Data Type Conversion24/1 -> Bus Creator/25  "isAbleToCompleteTask_1"
  Data Type Conversion25/1 -> Bus Creator/26  "remainDistToGo_m"
  Data Type Conversion26/1 -> Bus Creator/27  "remainTimeToSpend_sec"
  Data Type Conversion27/1 -> Bus Creator/28  "remainPowerWhenFinish_per"
  Data Type Conversion28/1 -> Bus Creator/29  "airSpeedCmd_ms"
  Data Type Conversion29/1 -> Bus Creator/30  "dheight_ms"
  [Vd_ms] -> Display/1, Data Type Conversion29/1
  Bus Selector/19 -> Selector/1  "<curVelNED>"
  Selector/1 -> Gain/1
  Gain/1 -> [Vd_ms]
  Demux2/3 -> Display1/1, Scope/1, [curHeightFromHome_m]
  Saturation/1 -> Data Type Conversion3/1
  MATLAB Function2/1(out) -> Display2/1, Scope1/1, Data Type Conversion/1
  Weighted Sample Time/1 -> MATLAB Function2/1(Ts)
  In3/1 -> Rate Transition/1
  Bus Selector2/1 -> Abs/1  "<windSpeed_ms>"
  Rate Transition/1 -> Bus Selector2/1
  From29/1 -> MATLAB Function4/1(windspeed_ms)
  Abs/1 -> [windSpeed_ms]

== system RefModel_SystemArchitecture/FlightControlFirmware/Controller/Subsystem ==
  In1 : Inport
  Bus Creator : BusCreator  Inputs=5  OutDataTypeStr=Bus: BUS_CTRL_dbg_param
      settings: InheritFromInputs=off
  Bus Selector1 : BusSelector  OutputSignals=mavlink_ctrl_param.headingCmd,mavlink_ctrl_param.groundspeedCmd,mavlink_ctrl_param.heightCmd,mavlink_ctrl_param.flightTaskMode,mavlink_ctrl_param.maxClimbSpeed
  Out1 : Outport
  wires:
  Bus Selector1/1 -> Bus Creator/1  "<headingCmd>"
  Bus Creator/1 -> Out1/1
  In1/1 -> Bus Selector1/1
  Bus Selector1/2 -> Bus Creator/2  "<groundspeedCmd>"
  Bus Selector1/3 -> Bus Creator/3  "<heightCmd>"
  Bus Selector1/4 -> Bus Creator/4  "<flightTaskMode>"
  Bus Selector1/5 -> Bus Creator/5  "<maxClimbSpeed>"

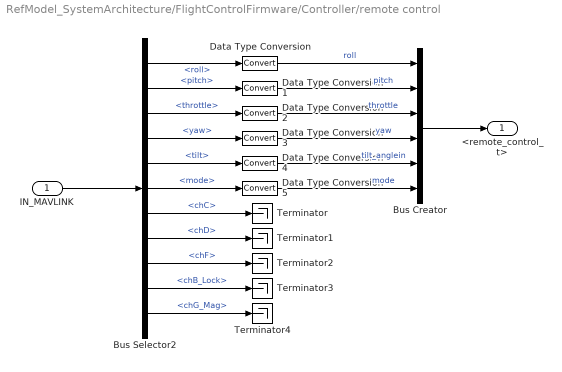
== system RefModel_SystemArchitecture/FlightControlFirmware/Controller/remote control ==
  IN_MAVLINK : Inport
  Bus Creator : BusCreator  Inputs=6  OutDataTypeStr=Bus: BUS_CTRL_remote_ct_st  NonVirtualBus=on
      settings: InheritFromInputs=off
  Bus Selector2 : BusSelector  OutputSignals=remote_control_t.roll,remote_control_t.pitch,remote_control_t.throttle,remote_control_t.yaw,remote_control_t.tilt,remote_control_t.mode,remote_control_t.chC,remote_control_t.chD,remote_control_t.chF,remote_control_t.chB_Lock,remote_control_t.chG_Mag
  Data Type Conversion{,1..5} (6 alike) : DataTypeConversion
  Terminator{,1..4} (5 alike) : Terminator
  <remote_control_t> : Outport
  wires:
  IN_MAVLINK/1 -> Bus Selector2/1
  Bus Creator/1 -> <remote_control_t>/1
  Bus Selector2/1 -> Data Type Conversion/1  "<roll>"
  Bus Selector2/2 -> Data Type Conversion1/1  "<pitch>"
  Bus Selector2/3 -> Data Type Conversion2/1  "<throttle>"
  Bus Selector2/4 -> Data Type Conversion3/1  "<yaw>"
  Bus Selector2/5 -> Data Type Conversion4/1  "<tilt>"
  Bus Selector2/6 -> Data Type Conversion5/1  "<mode>"
  Data Type Conversion/1 -> Bus Creator/1  "roll"
  Data Type Conversion1/1 -> Bus Creator/2  "pitch"
  Data Type Conversion2/1 -> Bus Creator/3  "throttle"
  Data Type Conversion3/1 -> Bus Creator/4  "yaw"
  Data Type Conversion4/1 -> Bus Creator/5  "tilt_anglein"
  Data Type Conversion5/1 -> Bus Creator/6  "mode"
  Bus Selector2/7 -> Terminator/1  "<chC>"
  Bus Selector2/8 -> Terminator1/1  "<chD>"
  Bus Selector2/9 -> Terminator2/1  "<chF>"
  Bus Selector2/10 -> Terminator3/1  "<chB_Lock>"
  Bus Selector2/11 -> Terminator4/1  "<chG_Mag>"

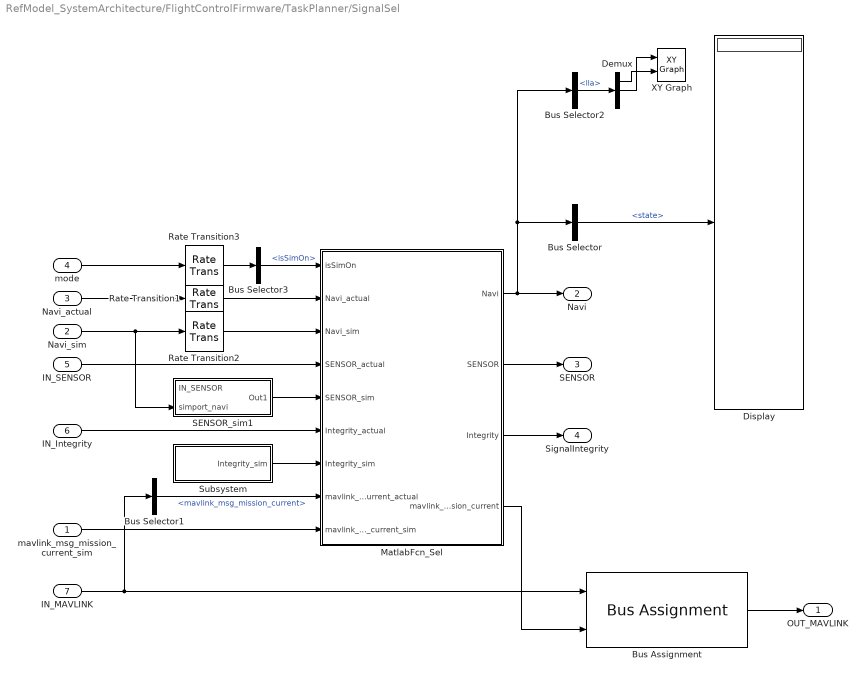
== system RefModel_SystemArchitecture/FlightControlFirmware/TaskPlanner/SignalSel ==
  mavlink_msg_mission_current_sim : Inport
  Navi_sim : Inport  Port=2
  Navi_actual : Inport  Port=3
  mode : Inport  Port=4
  IN_SENSOR : Inport  Port=5
  IN_Integrity : Inport  Port=6
  IN_MAVLINK : Inport  Port=7
  Bus Assignment : BusAssignment  AssignedSignals=mavlink_msg_mission_current
  Bus Selector : BusSelector  OutputSignals=state
  Bus Selector1 : BusSelector  OutputSignals=mavlink_msg_mission_current
  Bus Selector2 : BusSelector  OutputSignals=lla
  Bus Selector3 : BusSelector  OutputSignals=isSimOn
  Demux : Demux  Outputs=3
  Display : Display
  MatlabFcn_Sel : MATLAB Function  TreatAsAtomicUnit=on
  Rate Transition1 : RateTransition
  Rate Transition2 : RateTransition
  Rate Transition3 : RateTransition
  SENSOR_sim1 : Subsystem
  Subsystem : Subsystem
  XY Graph : simulink/Sinks/XY Graph  xmin=116.34  xmax=116.42  ymin=40.02  ymax=40.08  st=-1
  OUT_MAVLINK : Outport
  Navi : Outport  Port=2
  SENSOR : Outport  Port=3
  SignalIntegrity : Outport  Port=4
  wires:
  Navi_actual/1 -> Rate Transition1/1
  Navi_sim/1 -> SENSOR_sim1/2(simport_navi), Rate Transition2/1
  mode/1 -> Rate Transition3/1
  Rate Transition1/1 -> MatlabFcn_Sel/2(Navi_actual)
  Bus Selector3/1 -> MatlabFcn_Sel/1(isSimOn)  "<isSimOn>"
  Rate Transition3/1 -> Bus Selector3/1
  Rate Transition2/1 -> MatlabFcn_Sel/3(Navi_sim)
  MatlabFcn_Sel/1(Navi) -> Navi/1, Bus Selector2/1, Bus Selector/1
  Bus Selector/1 -> Display/1  "<state>"
  IN_SENSOR/1 -> MatlabFcn_Sel/4(SENSOR_actual)
  SENSOR_sim1/1(Out1) -> MatlabFcn_Sel/5(SENSOR_sim)
  IN_Integrity/1 -> MatlabFcn_Sel/6(Integrity_actual)
  Subsystem/1(Integrity_sim) -> MatlabFcn_Sel/7(Integrity_sim)
  MatlabFcn_Sel/2(SENSOR) -> SENSOR/1
  MatlabFcn_Sel/3(Integrity) -> SignalIntegrity/1
  IN_MAVLINK/1 -> Bus Selector1/1, Bus Assignment/1
  Bus Assignment/1 -> OUT_MAVLINK/1
  Bus Selector1/1 -> MatlabFcn_Sel/8(mavlink_msg_mission_current_actual)  "<mavlink_msg_mission_current>"
  mavlink_msg_mission_current_sim/1 -> MatlabFcn_Sel/9(mavlink_msg_mission_current_sim)
  MatlabFcn_Sel/4(mavlink_msg_mission_current) -> Bus Assignment/2
  Bus Selector2/1 -> Demux/1  "<lla>"
  Demux/2 -> XY Graph/1
  Demux/1 -> XY Graph/2

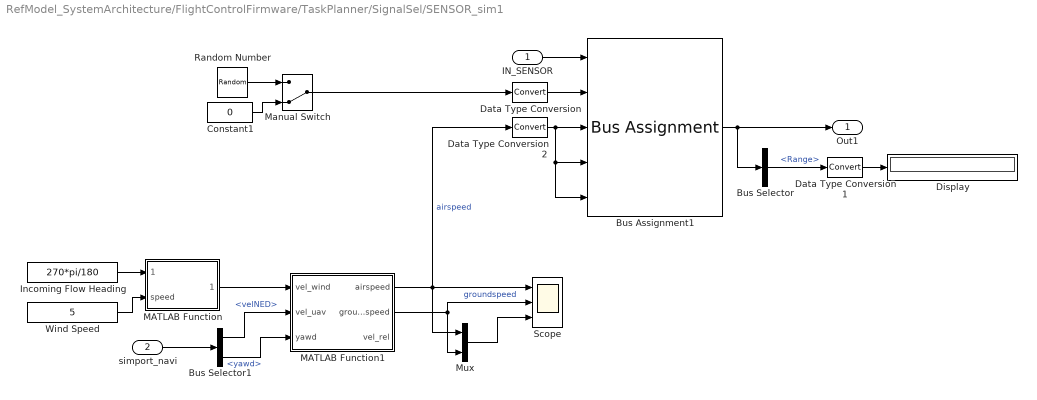
== system RefModel_SystemArchitecture/FlightControlFirmware/TaskPlanner/SignalSel/SENSOR_sim1 ==
  IN_SENSOR : Inport  OutDataTypeStr=Bus: BUS_SENSOR  BusOutputAsStruct=on
  simport_navi : Inport  Port=2
  Bus Assignment1 : BusAssignment  AssignedSignals=radar1.Range,airspeed1.airspeed,airspeed1.airspeed_true,airspeed1.airspeed_indicate
  Bus Selector : BusSelector  OutputSignals=radar1.Range
  Bus Selector1 : BusSelector  OutputSignals=velNED,yawd
  Constant1 : Constant  Value=0
  Data Type Conversion : DataTypeConversion
  Data Type Conversion1 : DataTypeConversion
  Data Type Conversion2 : DataTypeConversion
  Display : Display
  Incoming Flow Heading : Constant  Value=270*pi/180
  MATLAB Function : MATLAB Function  TreatAsAtomicUnit=on
  MATLAB Function1 : MATLAB Function  TreatAsAtomicUnit=on
  Manual Switch : ManualSwitch  CurrentSetting=0
  Mux : Mux  Inputs=2
  Random Number : RandomNumber
  Scope : Scope  NumInputPorts=3
  Wind Speed : Constant  Value=5
  Out1 : Outport
  wires:
  Constant1/1 -> Manual Switch/2
  Bus Assignment1/1 -> Bus Selector/1, Out1/1
  Data Type Conversion2/1 -> Bus Assignment1/5, Bus Assignment1/4, Bus Assignment1/3
  Bus Selector1/2 -> MATLAB Function1/3(yawd)  "<yawd>"
  Data Type Conversion/1 -> Bus Assignment1/2
  Incoming Flow Heading/1 -> MATLAB Function/1(heading)
  IN_SENSOR/1 -> Bus Assignment1/1
  Mux/1 -> Scope/3
  Manual Switch/1 -> Data Type Conversion/1
  Bus Selector1/1 -> MATLAB Function1/2(vel_uav)  "<velNED>"
  simport_navi/1 -> Bus Selector1/1
  Random Number/1 -> Manual Switch/1
  MATLAB Function/1(velNED_wind) -> MATLAB Function1/1(vel_wind)
  Data Type Conversion1/1 -> Display/1
  Wind Speed/1 -> MATLAB Function/2(speed)
  MATLAB Function1/1(airspeed) -> Data Type Conversion2/1, Scope/1, Mux/1  "airspeed"
  MATLAB Function1/2(groundspeed) -> Mux/2, Scope/2  "groundspeed"
  Bus Selector/1 -> Data Type Conversion1/1  "<Range>"

== system RefModel_SystemArchitecture/FlightControlFirmware/TaskPlanner/SignalSel/Subsystem ==
  Bus Assignment1 : BusAssignment  AssignedSignals=SystemHealthStatus
  Constant : Constant  Value=ENUM_SystemHealthStatus.SystemHealth  OutDataTypeStr=Enum: ENUM_SystemHealthStatus
  Constant1 : Constant  Value=ENUM_SystemHealthStatus.CanNotFly  OutDataTypeStr=Enum: ENUM_SystemHealthStatus
  Constant2 : Constant  Value=0  OutDataTypeStr=Bus: BUS_NAVI_SensorSignalIntegrity
  Manual Switch : ManualSwitch
  Integrity_sim : Outport
  wires:
  Bus Assignment1/1 -> Integrity_sim/1
  Constant1/1 -> Manual Switch/2
  Manual Switch/1 -> Bus Assignment1/2
  Constant/1 -> Manual Switch/1
  Constant2/1 -> Bus Assignment1/1

== matlab function RefModel_SystemArchitecture/FlightControlFirmware/TaskPlanner/SignalSel/SENSOR_sim1/MATLAB Function ==
  data: heading input; velNED_wind output; speed input
function velNED_wind = fcn(heading,speed)
velNED_wind = speed*[cos(heading);sin(heading);0];

== matlab function RefModel_SystemArchitecture/FlightControlFirmware/datatype3/MATLAB Function ==
  data: u input; u output
function u = fcn(u)
u = rem(u,2*pi);
if u > pi
    u = u - 2*pi;
end

== matlab function RefModel_SystemArchitecture/FlightControlFirmware/TaskPlanner/SignalSel/SENSOR_sim1/MATLAB Function1 ==
  data: vel_wind input; airspeed output; groundspeed output; vel_uav input; vel_rel output; yawd input
function [airspeed,groundspeed,vel_rel] = fcn(vel_wind,vel_uav, yawd)
vel_rel = vel_wind + vel_uav;
airspeedNorm = norm(vel_rel(1:2));
windInc = atan2(vel_wind(2),vel_wind(1));
dyaw = angdiff(yawd*pi/180,windInc);
windvel_alongheading = cos(dyaw)*norm(vel_wind(1:2));
airspeed = norm(vel_uav(1:2)) + windvel_alongheading;
% airspeed = airspeedNorm;
groundspeed = norm(vel_uav(1:2));
% fprintf('airspeed:%.0f,airspeed1:%.0f\n',airspeed,airspeed1)

== matlab function RefModel_SystemArchitecture/FlightControlFirmware/TaskPlanner/SignalSel/MatlabFcn_Sel ==
  data: isSimOn input; Navi output Bus: BUS_NAVI_TO_FIRM size=1; Navi_actual input Bus: BUS_NAVI_TO_FIRM size=1; Navi_sim input Bus: BUS_NAVI_TO_FIRM size=1; SENSOR_actual input Bus: BUS_SENSOR; SENSOR_sim input Bus: BUS_SENSOR; Integrity_actual input Bus: BUS_NAVI_SensorSignalIntegrity; Integrity_sim input Bus: BUS_NAVI_SensorSignalIntegrity; SENSOR output Bus: BUS_SENSOR; Integrity output Bus: BUS_NAVI_SensorSignalIntegrity; mavlink_msg_mission_current_actual input Bus: mavlink_msg_mission_current size=3; mavlink_msg_mission_current_sim input Bus: mavlink_msg_mission_current size=3; mavlink_msg_mission_current output Bus: mavlink_msg_mission_current size=3
function [Navi,SENSOR,Integrity,mavlink_msg_mission_current] = fcn(isSimOn,Navi_actual,Navi_sim, SENSOR_actual, SENSOR_sim, Integrity_actual, Integrity_sim, mavlink_msg_mission_current_actual,mavlink_msg_mission_current_sim)
persistent simStatus
if isempty(simStatus)
    simStatus = isSimOn;
end
if isSimOn
    Navi = Navi_sim;
    SENSOR = SENSOR_sim;
    Integrity = Integrity_sim;
    mavlink_msg_mission_current = mavlink_msg_mission_current_sim;
else
    Navi = Navi_actual;
    SENSOR = SENSOR_actual;
    Integrity = Integrity_actual;    
    mavlink_msg_mission_current = mavlink_msg_mission_current_actual;
end
if isSimOn == 1
    sl = 1;
end
if simStatus ~= isSimOn
    if isSimOn
        fprintf('Switch To Task Simulation Mode!\n');
    else
        fprintf('Switch To Normal Mode!\n');
    end
end
simStatus = isSimOn;

== matlab function RefModel_SystemArchitecture/FlightControlFirmware/datatype3/MATLAB Function1 ==
  data: u input; u output
function u = fcn(u)
u = rem(u,2*pi);
if u > pi
    u = u - 2*pi;
elseif u < -pi
    u = u + 2*pi;
end

== matlab function RefModel_SystemArchitecture/FlightControlFirmware/datatype3/MATLAB Function2 ==
  data: Ts input; u input; out output; taskmode input; uavmode input
function out = fcn(Ts, u,taskmode,uavmode)
persistent preUavMode count1 count2 becomeFix becomeRotor preout
if isempty(preUavMode)
    preUavMode = uavmode;
    count1 = 0;
    count2 = 0;
    becomeFix = false;
    becomeRotor = false;
    preout = 0;
end
timeToWait = 5;
if (preUavMode == ENUM_UAVMode.Fix2Rotor || preUavMode == ENUM_UAVMode.Fix) && ...
        uavmode == ENUM_UAVMode.Rotor
    becomeRotor = true;
    count2 = 0;
else
    count2 = count2 + Ts;
    if count2 > timeToWait
        becomeRotor = false;
    end
end
if preUavMode == ENUM_UAVMode.Rotor2Fix && ...
        uavmode == ENUM_UAVMode.Fix
    becomeFix = true;
    count1 = 0;
else
    count1 = count1 + Ts;
    if count1 > timeToWait
        becomeFix = false;
    end
end
preUavMode = uavmode;
out = u;
switch taskmode
    case ENUM_FlightTaskMode.GoHomeMode
        out = 1001; % 正在返航
    case {ENUM_FlightTaskMode.HoverAdjustMode,...
            ENUM_FlightTaskMode.AirStandByMode}
        if preout == 1503 % 前一时刻out值为"已切换到旋翼"
            out = 1503;
        else
            out = 1004; % 悬停中                                 
        end
    case ENUM_FlightTaskMode.TakeOffMode
        out = 1005; % 爬升
    case ENUM_FlightTaskMode.LandMode
        out = 1007; % 着陆
    case ENUM_FlightTaskMode.HoverUpMode
        out = 1500; % 盘旋上升
    case ENUM_FlightTaskMode.HoverDownMode
        out = 1501; % 盘旋下降
    case ENUM_FlightTaskMode.Rotor2Fix_Mode
        out = 1504; % 切换固定翼
    case ENUM_FlightTaskMode.Fix2Rotor_Mode
        out = 1505; % 切换旋翼
end
if becomeFix
    out = 1502; % 已切换到固定翼
end
if becomeRotor
    out = 1503; % 已切换到旋翼 
end
preout = out;

== matlab function RefModel_SystemArchitecture/FlightControlFirmware/datatype3/MATLAB Function4 ==
  data: windspeed_ms input; warningFlag output
function warningFlag = fcn(windspeed_ms)
warningFlag = false(256,1);
%% 风相关
if isVeryHighWind(windspeed_ms)
    warningFlag(1) = true;
elseif isHighWind(windspeed_ms)
    warningFlag(2) = true;
end
%% 电池相关

 

function flag = isVeryHighWind(windspeed)
flag = false;
if windspeed > 13.8 % 6级风
    flag = true; 
end
function flag = isHighWind(windspeed)
flag = false;
if windspeed > 10 % 6级风
    flag = true; 
end

== matlab function RefModel_SystemArchitecture/FlightControlFirmware/Form_Debug_WarningInfo512/MATLAB Function3 ==
  data: u input; u output
function u = fcn(u)
u = max(0,u);

== matlab function RefModel_SystemArchitecture/FlightControlFirmware/Form_Debug_WarningInfo512/FormatWarning512 ==
  data: clock_sec input; Ts input; windspeed_ms input; warningFlag output; Task_RTInfo input Bus: BUS_TASK_RTInfo; TaskModeData input Bus: BUS_TASK_PATH_OutParam; SensorStatus input Bus: BUS_NAVI_SensorSignalIntegrity_Status; beforeTakeOff output; afterLand output
function [warningFlag,beforeTakeOff,afterLand]  = fcn(clock_sec, Ts, windspeed_ms, Task_RTInfo, TaskModeData, SensorStatus)
%% 
% 1. 空中风速过大,飞机将返航 (非地面模式播报)
% 2. 空中风速很大,需谨慎 (非地面模式播报)
% 3. 电池严重低电量,飞机将立即降落 (非地面模式播报)
% 4. 电池低电量,飞机将返航 (非地面模式播报)
% 5. 通信失联,飞机将返航 (非地面模式播报)
% 6. 超出电子围栏,飞机将返航 (非地面模式播报)
% 7. 进入失速,飞机将转旋翼并返航 (非地面模式播报)
% 8. 飞机从失速中恢复,将以返航 (非地面模式播报)
% 9. 传感器系统可用性降级,飞机将返航 (非地面模式播报)
% 10.传感器系统故障,飞机将立即降落 (非地面模式播报)
% 11.检测到下方近距离有物体,飞机将在当前高度切换旋翼 (非地面模式播报)
% 12.导航数据不可用,GPS或磁力计可能受到干扰,飞机可能无法解锁或起飞,若重启后该故障若仍然存在，请联系厂家 (仅地面模式播报)
% 13.航点无效,飞机禁止起飞，重新启动飞机并设置航点
% 14.检测到磁场异常,飞机可能无法解锁或起飞,若重启后该故障若仍然存在，请联系厂家 (仅地面模式播报)
% 15.传感器系统可用性降级或故障，点击起飞后飞机将自动加锁,若重启后该故障若仍然存在，请联系厂家 (仅地面模式播报)
% 16.飞行中检测到异常的大姿态运动，飞机将返航 (非地面模式播报)
persistent flagHasTakeOff flagHasLand
if isempty(flagHasTakeOff)
    flagHasTakeOff = false;
    flagHasLand = false;
end
if TaskModeData.flightTaskMode == ENUM_FlightTaskMode.TakeOffMode
    flagHasTakeOff = true;
end
if TaskModeData.flightTaskMode == ENUM_FlightTaskMode.LandMode
    flagHasLand = true;
end
afterTakeOff = flagHasTakeOff;
beforeTakeOff = TaskModeData.flightTaskMode == ENUM_FlightTaskMode.GroundStandByMode && ~flagHasTakeOff;
afterLand = TaskModeData.flightTaskMode == ENUM_FlightTaskMode.GroundStandByMode && flagHasLand;
warningFlag = false(512,1);
if clock_sec < 60
    return;
end
%% 风相关
if TaskModeData.flightTaskMode ~= ENUM_FlightTaskMode.GroundStandByMode
    if isVeryHighWind(windspeed_ms)
        % 非常大风
        warningFlag(1) = true;
        %     warningFlag(2) = true;
    else
        if isHighWind(windspeed_ms)
            % 大风
            warningFlag(2) = true;
        end
    end
end
%% 电池相关
if TaskModeData.flightTaskMode ~= ENUM_FlightTaskMode.GroundStandByMode
    if Task_RTInfo.BatteryStatus == ENUM_BatteryStatus.BatterySevereLow
        % 电池严重低电量
        warningFlag(3) = true;
    %     warningFlag(4) = true;
    else
        if Task_RTInfo.BatteryStatus == ENUM_BatteryStatus.BatteryLow
            % 电池低电量
            warningFlag(4) = true;
        end
    end
end
%% 通信
if TaskModeData.flightTaskMode ~= ENUM_FlightTaskMode.GroundStandByMode
    if Task_RTInfo.ComStatus == ENUM_ComStatus.RemoteOrStationLost
        % 通信失联
        warningFlag(5) = true;
    end
end
%% 电子栅栏
if TaskModeData.flightTaskMode ~= ENUM_FlightTaskMode.GroundStandByMode
    if Task_RTInfo.FenseStatus == ENUM_RTInfo_Fense.FenseStatus_Out
        % 超出电子围栏
        warningFlag(6) = true;
    end
end
%% 失速
if TaskModeData.flightTaskMode ~= ENUM_FlightTaskMode.GroundStandByMode
    if Task_RTInfo.StallStatus == ENUM_RTInfo_Stall.StallStatus_InStall
        % 进入失速
        warningFlag(7) = true;
    elseif Task_RTInfo.StallStatus == ENUM_RTInfo_Stall.StallStatus_Recovery
        % 从失速中恢复
        warningFlag(8) = true;    
    end
end
%% 传感器系统健康度
if TaskModeData.flightTaskMode ~= ENUM_FlightTaskMode.GroundStandByMode
    if Task_RTInfo.SensorStatus == ENUM_RTInfo_SensorHealth.SensorRT_Degrade
        % 传感器系统可用性降级,飞机将返航
        warningFlag(9) = true;    
    elseif Task_RTInfo.SensorStatus == ENUM_RTInfo_SensorHealth.SensorRT_Fault
        % 传感器系统故障,飞机将立即降落
        warningFlag(10) = true;
    end
else
    if Task_RTInfo.SensorStatus == ENUM_RTInfo_SensorHealth.SensorRT_Degrade || ...
            Task_RTInfo.SensorStatus == ENUM_RTInfo_SensorHealth.SensorRT_Fault
        % 传感器系统可用性降级或故障，点击起飞后飞机将自动加锁，,若重启后该故障若仍然存在，请联系厂家
        warningFlag(15) = true;
    end
end
%% 固定翼高度
if TaskModeData.flightTaskMode ~= ENUM_FlightTaskMode.GroundStandByMode
    if Task_RTInfo.FixWingHeightStatus == ENUM_RTInfo_FixHeight.FixWingHeight_TooLow
        % 固定翼模式下检测到下方近距离有物体
        warningFlag(11) = true;
    end
end
%% 组合导航有效性
if beforeTakeOff && clock_sec > 360
    if Task_RTInfo.NaviStatus ~= ENUM_NaviStatus.NaviNormal
        % 导航数据不可用,若重启后该故障若仍然存在，请联系厂家
        warningFlag(12) = true;    
    end
end
%% 航点有效性
if Task_RTInfo.Warning == ENUM_RTInfo_Warn.Warn_Path_Not_Valid
    % 航点无效，飞机禁止起飞，重新重启飞机并设置航点
%     warningFlag(13) = true;    
end
%% 磁力计异常
% 检测到磁场异常,禁止起飞,若重启后该故障若仍然存在，请联系厂家
if beforeTakeOff 
    warningFlag(14) = isAllMagFault(flagHasTakeOff,SensorStatus,Ts,clock_sec);
end
%% 大姿态异常
if TaskModeData.flightTaskMode ~= ENUM_FlightTaskMode.GroundStandByMode 
    if Task_RTInfo.AttitudeStatus == ENUM_RTInfo_LargeAttitude.LargeAttitude_Abnormal
        % 飞行中检测到异常的大姿态运动，飞机将返航
        warningFlag(16) = true;
    end
end
%% ----------------------------------------------------------------------------
function flag = isVeryHighWind(windspeed)
flag = false;
if windspeed > 13.8 % 6级风
    flag = true; 
end
function flag = isHighWind(windspeed)
flag = false;
if windspeed > 10 % 6级风
    flag = true; 
end
function flag = isAllMagFault(flagHasTakeOff,SensorStatus,Ts,clock_sec)
persistent du
if isempty(du)
    du = 0; 
end
flag = false;
if clock_sec > 60 && ... % 开机后一段时间后开始生效
    ~flagHasTakeOff && ...% 仅在地面模式生效
        (SensorStatus.mag1 ~= ENUM_SensorHealthStatus.Health && SensorStatus.mag2 ~= ENUM_SensorHealthStatus.Health)
    du = du + Ts;
    if du > 5 % 
        fprintf('\n');
        flag = true;
    end
else
    du = 0;
end
